simulink model "controller_hor"  (R2020b)
settings: Solver=ode45  StartTime=0.0  StopTime=2  MaxStep=0.01  RelTol=1e-3
values from neighbouring files (symbols this model uses):
  g = 9.81    [matlab.mat]
  J_xx = 400    [matlab.mat]
  J_yy = 1    [matlab.mat]
  J_zz = 400    [matlab.mat]
  k_f = 6.11e-08    [matlab.mat]
  l = 400    [matlab.mat]
  m = 1.5    [matlab.mat]
  time = 25    [matlab.mat]
  x_0 = 0    [matlab.mat]
  x_des = 6    [matlab.mat]
  y_0 = 0    [matlab.mat]
  y_des = 6    [matlab.mat]
  z_0 = 0    [matlab.mat]
  z_des = 6    [matlab.mat]
undefined symbols (not defined in the file or in its folder): k_p_fi, k_p_psi, k_p_theta, k_p_x, k_p_y, k_p_z, k_v_fi, k_v_psi, k_v_theta, k_v_x, k_v_y, k_v_z, k_X, k_Y, x_dot_min
settings Model: OrderedModelArguments=off  Creator=Danil  LastModifiedBy=Danil
settings DataIOCC: ReturnWorkspaceOutputsName=SDOSimTest_Log

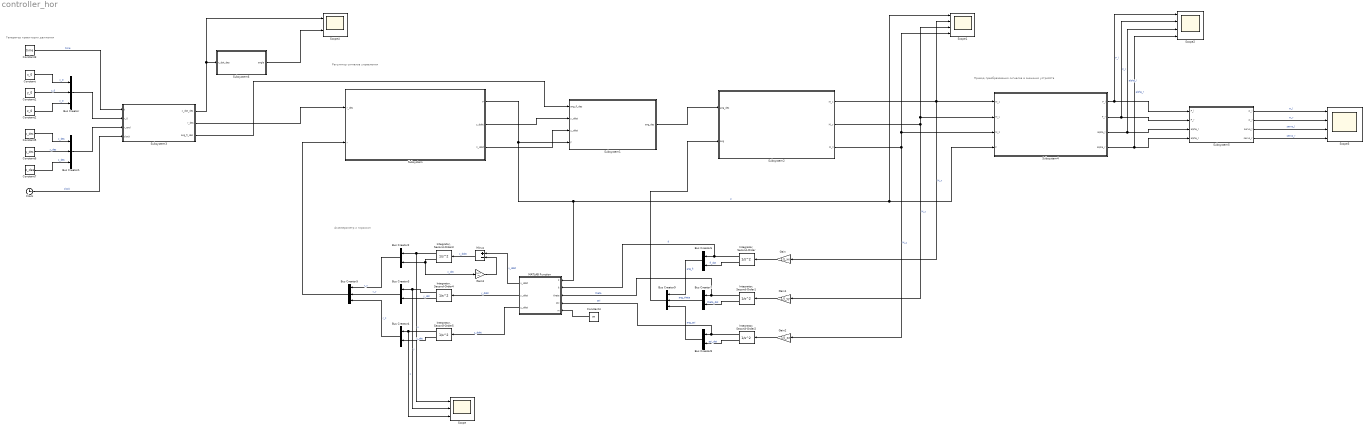
== system controller_hor ==
  note: Привод преобразования сигналов в значения устройств
  note: Регулятор сигналов управления
  note: Генератор траектории движения
  note: Акселерометр и гироскоп
  Bus Creator{,1,5,9} (4 alike) : BusCreator  Inputs=3
  Bus Creator{2..4,6..8} (6 alike) : BusCreator  Inputs=2
  Clock : Clock
  Constant : Constant  Value=x_0
  Constant1 : Constant  Value=y_0
  Constant2 : Constant  Value=z_0
  Constant3 : Constant  Value=time
  Constant4 : Constant  Value=m
  Constant5 : Constant  Value=x_des
  Constant6 : Constant  Value=y_des
  Constant7 : Constant  Value=z_des
  Gain : Gain  Gain=1/J_xx
  Gain1 : Gain  Gain=1/J_yy
  Gain2 : Gain  Gain=1/J_zz
  Gain3 : Gain  Gain=k_X / m
  Integrator, Second-Order{,1..2,4..5} (5 alike) : SecondOrderIntegrator
  "Integrator, Second-Order3" : SecondOrderIntegrator  ICDXDT=x_dot_min
  MATLAB Function : MATLAB Function  TreatAsAtomicUnit=on
  Minus : Sum  Inputs=+-
  Scope : Scope  NumInputPorts=3
  Scope1 : Scope  NumInputPorts=4
  Scope2 : Scope  NumInputPorts=4
  Scope3 : Scope  NumInputPorts=4
  Scope4 : Scope  NumInputPorts=2
  Subsystem : Subsystem
  Subsystem1 : Subsystem
  Subsystem2 : Subsystem
  Subsystem3 : Subsystem
  Subsystem4 : Subsystem
  Subsystem5 : Subsystem
  Subsystem6 : Subsystem
  wires:
  Subsystem2/2(M_y) -> Gain1/1, Subsystem4/2(M_y), Scope1/3  "M_y"
  Constant2/1 -> Bus Creator/3  "z_0"
  Subsystem5/4(servo_r) -> Scope3/4  "servo_r"
  Subsystem2/1(M_x) -> Subsystem4/1(M_x), Gain/1, Scope1/2  "M_x"
  Subsystem4/2(F_r) -> Scope2/2, Subsystem5/2(F_r)  "F_r"
  Subsystem5/3(servo_l) -> Scope3/3  "servo_l"
  Subsystem5/1(w_l) -> Scope3/1  "w_l"
  Subsystem/2(y_ddot) -> Subsystem1/2(y_ddot)
  Bus Creator6/1 -> Bus Creator9/1  "ang_fi"
  Subsystem5/2(w_r) -> Scope3/2  "w_r"
  Subsystem4/4(alpha_r) -> Scope2/4, Subsystem5/4(alpha_r)  "alpha_r"
  Constant1/1 -> Bus Creator/2  "y_0"
  Subsystem4/3(alpha_l) -> Scope2/3, Subsystem5/3(alpha_l)  "alpha_l"
  "Integrator, Second-Order2"/2 -> Bus Creator8/2  "psi_dot"
  "Integrator, Second-Order"/2 -> Bus Creator6/2  "fi_dot"
  Subsystem4/1(F_l) -> Scope2/1, Subsystem5/1(F_l)  "F_l"
  "Integrator, Second-Order3"/1 -> Scope/1, Bus Creator2/1  "x"
  "Integrator, Second-Order5"/2 -> Bus Creator4/2  "z_dot"
  Constant4/1 -> MATLAB Function/5(m)
  "Integrator, Second-Order1"/1 -> MATLAB Function/3(theta), Bus Creator7/1  "theta"
  "Integrator, Second-Order1"/2 -> Bus Creator7/2  "theta_dot"
  Subsystem/1(F) -> Subsystem1/4(F), MATLAB Function/1(F), Scope1/1, Subsystem4/4(F)  "F"
  "Integrator, Second-Order2"/1 -> MATLAB Function/4(psi), Bus Creator8/1  "psi"
  Bus Creator7/1 -> Bus Creator9/2  "ang_theta"
  Gain2/1 -> "Integrator, Second-Order2"/1
  Subsystem/3(z_ddot) -> Subsystem1/3(z_ddot)
  Constant5/1 -> Bus Creator1/1  "x_des"
  Bus Creator4/1 -> Bus Creator5/3  "r_z"
  Bus Creator3/1 -> Bus Creator5/2  "r_y"
  Subsystem2/3(M_z) -> Gain2/1, Subsystem4/3(M_z), Scope1/4  "M_z"
  "Integrator, Second-Order"/1 -> MATLAB Function/2(fi), Bus Creator6/1  "fi"
  "Integrator, Second-Order4"/1 -> Scope/2, Bus Creator3/1  "y"
  Subsystem3/2(r_des) -> Subsystem/1(r_des)
  Subsystem3/3(ang_fi_des) -> Subsystem1/1(ang_fi_des)
  Constant7/1 -> Bus Creator1/3  "z_des"
  Bus Creator/1 -> Subsystem3/2(r_0)
  Constant3/1 -> Subsystem3/1(t)  "time"
  "Integrator, Second-Order3"/2 -> Gain3/1, Bus Creator2/2  "x_dot"
  Bus Creator2/1 -> Bus Creator5/1  "r_x"
  Bus Creator5/1 -> Subsystem/2(r)
  "Integrator, Second-Order4"/2 -> Bus Creator3/2  "y_dot"
  MATLAB Function/3(z_ddot) -> "Integrator, Second-Order5"/1  "z_ddot"
  Clock/1 -> Subsystem3/4(clock)  "clock"
  Bus Creator1/1 -> Subsystem3/3(r_end)
  "Integrator, Second-Order5"/1 -> Scope/3, Bus Creator4/1  "z"
  Constant/1 -> Bus Creator/1  "x_0"
  Gain1/1 -> "Integrator, Second-Order1"/1
  MATLAB Function/2(y_ddot) -> "Integrator, Second-Order4"/1  "y_ddot"
  Bus Creator8/1 -> Bus Creator9/3  "ang_psi"
  Gain/1 -> "Integrator, Second-Order"/1
  Constant6/1 -> Bus Creator1/2  "y_des"
  Subsystem3/1(x_dot_des) -> Scope4/1, Subsystem6/1(x_dot_des)
  Subsystem1/1(ang_des) -> Subsystem2/1(ang_des)
  Bus Creator9/1 -> Subsystem2/2(ang)
  Subsystem6/1(angle) -> Scope4/2
  Minus/1 -> "Integrator, Second-Order3"/1  "x_ddot"
  MATLAB Function/1(x_ddot) -> Minus/1  "x_ddot"
  Gain3/1 -> Minus/2

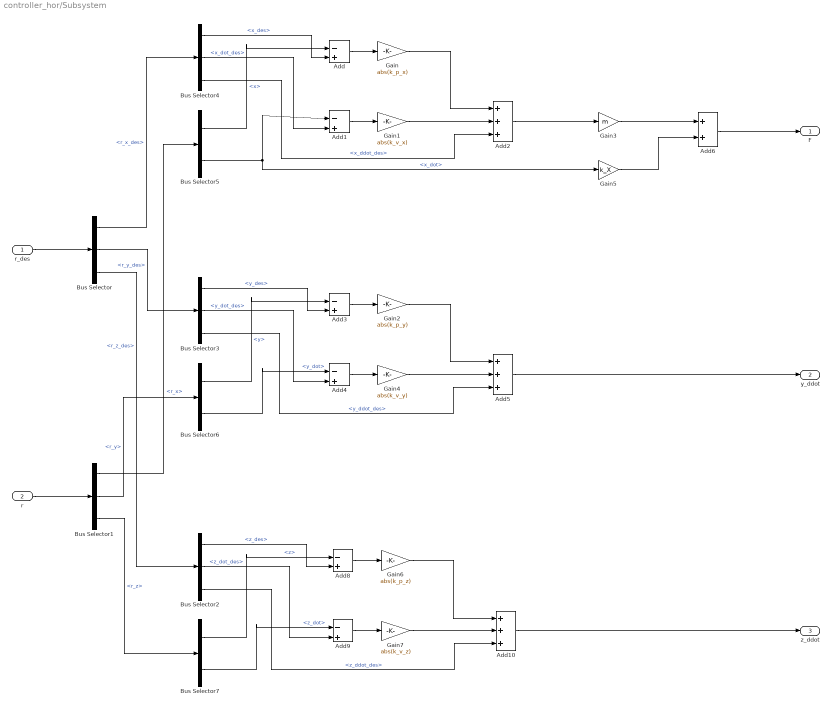
== system controller_hor/Subsystem ==
  r_des : Inport
  r : Inport  Port=2
  Add{,1,3..4,8..9} (6 alike) : Sum  Inputs=-|+
  Add10 : Sum  Inputs=+++
  Add2 : Sum  Inputs=+++
  Add5 : Sum  Inputs=+++
  Add6 : Sum
  Bus Selector : BusSelector  OutputSignals=r_x_des,r_y_des,r_z_des
  Bus Selector1 : BusSelector  OutputSignals=r_x,r_y,r_z
  Bus Selector2 : BusSelector  OutputSignals=z_des,z_dot_des,z_ddot_des
  Bus Selector3 : BusSelector  OutputSignals=y_des,y_dot_des,y_ddot_des
  Bus Selector4 : BusSelector  OutputSignals=x_des,x_dot_des,x_ddot_des
  Bus Selector5 : BusSelector  OutputSignals=x,x_dot
  Bus Selector6 : BusSelector  OutputSignals=y,y_dot
  Bus Selector7 : BusSelector  OutputSignals=z,z_dot
  Gain : Gain  Gain=abs(k_p_x)
  Gain1 : Gain  Gain=abs(k_v_x)
  Gain2 : Gain  Gain=abs(k_p_y)
  Gain3 : Gain  Gain=m
  Gain4 : Gain  Gain=abs(k_v_y)
  Gain5 : Gain  Gain=k_X
  Gain6 : Gain  Gain=abs(k_p_z)
  Gain7 : Gain  Gain=abs(k_v_z)
  F : Outport
  y_ddot : Outport  Port=2
  z_ddot : Outport  Port=3
  wires:
  Gain/1 -> Add2/1
  Add/1 -> Gain/1
  Add1/1 -> Gain1/1
  Gain1/1 -> Add2/2
  Add4/1 -> Gain4/1
  Add5/1 -> y_ddot/1
  Gain4/1 -> Add5/2
  Gain2/1 -> Add5/1
  Add3/1 -> Gain2/1
  Add9/1 -> Gain7/1
  Gain7/1 -> Add10/2
  Gain6/1 -> Add10/1
  Add8/1 -> Gain6/1
  Add10/1 -> z_ddot/1
  r_des/1 -> Bus Selector/1
  r/1 -> Bus Selector1/1
  Bus Selector4/1 -> Add/2  "<x_des>"
  Bus Selector4/2 -> Add1/2  "<x_dot_des>"
  Bus Selector4/3 -> Add2/3  "<x_ddot_des>"
  Bus Selector5/1 -> Add/1  "<x>"
  Bus Selector5/2 -> Gain5/1, Add1/1  "<x_dot>"
  Bus Selector3/1 -> Add3/2  "<y_des>"
  Bus Selector3/2 -> Add4/2  "<y_dot_des>"
  Bus Selector3/3 -> Add5/3  "<y_ddot_des>"
  Bus Selector6/1 -> Add3/1  "<y>"
  Bus Selector6/2 -> Add4/1  "<y_dot>"
  Bus Selector2/1 -> Add8/2  "<z_des>"
  Bus Selector2/2 -> Add9/2  "<z_dot_des>"
  Bus Selector2/3 -> Add10/3  "<z_ddot_des>"
  Bus Selector7/1 -> Add8/1  "<z>"
  Bus Selector7/2 -> Add9/1  "<z_dot>"
  Bus Selector/1 -> Bus Selector4/1  "<r_x_des>"
  Bus Selector/2 -> Bus Selector3/1  "<r_y_des>"
  Bus Selector/3 -> Bus Selector2/1  "<r_z_des>"
  Bus Selector1/1 -> Bus Selector5/1  "<r_x>"
  Bus Selector1/2 -> Bus Selector6/1  "<r_y>"
  Bus Selector1/3 -> Bus Selector7/1  "<r_z>"
  Add2/1 -> Gain3/1
  Gain3/1 -> Add6/1
  Add6/1 -> F/1
  Gain5/1 -> Add6/2

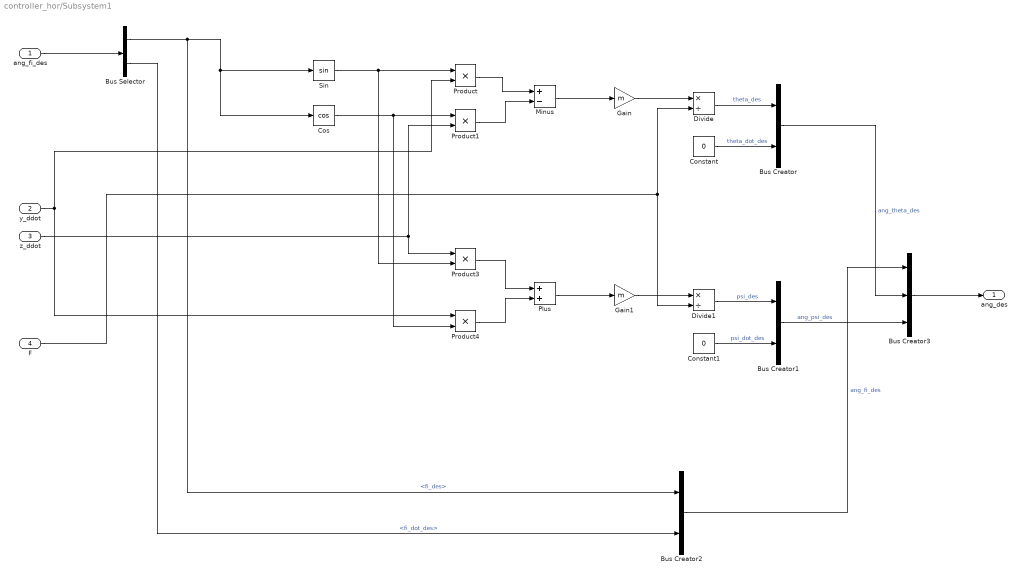
== system controller_hor/Subsystem1 ==
  ang_fi_des : Inport
  y_ddot : Inport  Port=2
  z_ddot : Inport  Port=3
  F : Inport  Port=4
  Bus Creator : BusCreator  Inputs=2
  Bus Creator1 : BusCreator  Inputs=2
  Bus Creator2 : BusCreator  Inputs=2
  Bus Creator3 : BusCreator  Inputs=3
  Bus Selector : BusSelector  OutputSignals=fi_des,fi_dot_des
  Constant : Constant  Value=0
  Constant1 : Constant  Value=0
  Cos : Trigonometry  Operator=cos
  Divide : Product  Inputs=*/
  Divide1 : Product  Inputs=*/
  Gain : Gain  Gain=m
  Gain1 : Gain  Gain=m
  Minus : Sum  Inputs=+-
  Plus : Sum
  Product{,1,3..4} (4 alike) : Product
  Sin : Trigonometry
  ang_des : Outport
  wires:
  Sin/1 -> Product3/2, Product/1
  Product1/1 -> Minus/2
  Product/1 -> Minus/1
  z_ddot/1 -> Product1/2, Product3/1
  Cos/1 -> Product4/2, Product1/1
  y_ddot/1 -> Product/2, Product4/1
  Product4/1 -> Plus/2
  Product3/1 -> Plus/1
  ang_fi_des/1 -> Bus Selector/1
  Bus Selector/1 -> Bus Creator2/1, Sin/1, Cos/1  "<fi_des>"
  Bus Selector/2 -> Bus Creator2/2  "<fi_dot_des>"
  Constant/1 -> Bus Creator/2  "theta_dot_des"
  Constant1/1 -> Bus Creator1/2  "psi_dot_des"
  Bus Creator3/1 -> ang_des/1
  Bus Creator2/1 -> Bus Creator3/1  "ang_fi_des"
  Minus/1 -> Gain/1
  Gain/1 -> Divide/1
  F/1 -> Divide/2, Divide1/2
  Divide/1 -> Bus Creator/1  "theta_des"
  Plus/1 -> Gain1/1
  Gain1/1 -> Divide1/1
  Divide1/1 -> Bus Creator1/1  "psi_des"
  Bus Creator/1 -> Bus Creator3/2  "ang_theta_des"
  Bus Creator1/1 -> Bus Creator3/3  "ang_psi_des"

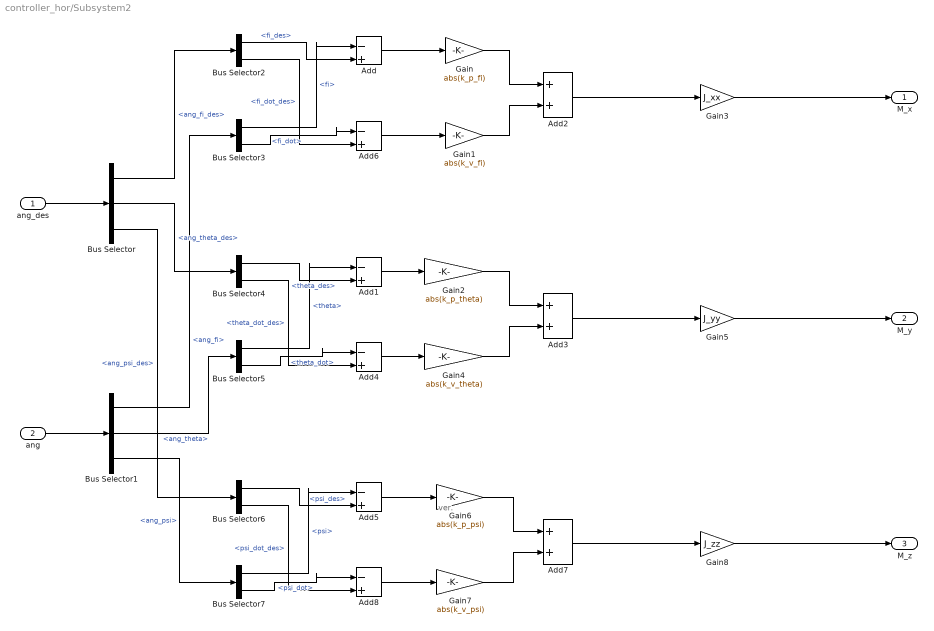
== system controller_hor/Subsystem2 ==
  note: ver.
  ang_des : Inport
  ang : Inport  Port=2
  Add{,1,4..6,8} (6 alike) : Sum  Inputs=-|+
  Add2 : Sum
  Add3 : Sum
  Add7 : Sum
  Bus Selector : BusSelector  OutputSignals=ang_fi_des,ang_theta_des,ang_psi_des
  Bus Selector1 : BusSelector  OutputSignals=ang_fi,ang_theta,ang_psi
  Bus Selector2 : BusSelector  OutputSignals=fi_des,fi_dot_des
  Bus Selector3 : BusSelector  OutputSignals=fi,fi_dot
  Bus Selector4 : BusSelector  OutputSignals=theta_des,theta_dot_des
  Bus Selector5 : BusSelector  OutputSignals=theta,theta_dot
  Bus Selector6 : BusSelector  OutputSignals=psi_des,psi_dot_des
  Bus Selector7 : BusSelector  OutputSignals=psi,psi_dot
  Gain : Gain  Gain=abs(k_p_fi)
  Gain1 : Gain  Gain=abs(k_v_fi)
  Gain2 : Gain  Gain=abs(k_p_theta)
  Gain3 : Gain  Gain=J_xx
  Gain4 : Gain  Gain=abs(k_v_theta)
  Gain5 : Gain  Gain=J_yy
  Gain6 : Gain  Gain=abs(k_p_psi)
  Gain7 : Gain  Gain=abs(k_v_psi)
  Gain8 : Gain  Gain=J_zz
  M_x : Outport
  M_y : Outport  Port=2
  M_z : Outport  Port=3
  wires:
  Gain/1 -> Add2/1
  Gain1/1 -> Add2/2
  Add/1 -> Gain/1
  Add2/1 -> Gain3/1
  Gain3/1 -> M_x/1
  Add6/1 -> Gain1/1
  Add1/1 -> Gain2/1
  Gain5/1 -> M_y/1
  Add3/1 -> Gain5/1
  Gain2/1 -> Add3/1
  Gain4/1 -> Add3/2
  Add4/1 -> Gain4/1
  Add5/1 -> Gain6/1
  Gain8/1 -> M_z/1
  Add7/1 -> Gain8/1
  Gain6/1 -> Add7/1
  Gain7/1 -> Add7/2
  Add8/1 -> Gain7/1
  ang_des/1 -> Bus Selector/1
  ang/1 -> Bus Selector1/1
  Bus Selector2/1 -> Add/2  "<fi_des>"
  Bus Selector3/1 -> Add/1  "<fi>"
  Bus Selector2/2 -> Add6/2  "<fi_dot_des>"
  Bus Selector3/2 -> Add6/1  "<fi_dot>"
  Bus Selector4/1 -> Add1/2  "<theta_des>"
  Bus Selector5/1 -> Add1/1  "<theta>"
  Bus Selector4/2 -> Add4/2  "<theta_dot_des>"
  Bus Selector5/2 -> Add4/1  "<theta_dot>"
  Bus Selector6/1 -> Add5/2  "<psi_des>"
  Bus Selector7/1 -> Add5/1  "<psi>"
  Bus Selector6/2 -> Add8/2  "<psi_dot_des>"
  Bus Selector7/2 -> Add8/1  "<psi_dot>"
  Bus Selector/1 -> Bus Selector2/1  "<ang_fi_des>"
  Bus Selector/2 -> Bus Selector4/1  "<ang_theta_des>"
  Bus Selector/3 -> Bus Selector6/1  "<ang_psi_des>"
  Bus Selector1/1 -> Bus Selector3/1  "<ang_fi>"
  Bus Selector1/2 -> Bus Selector5/1  "<ang_theta>"
  Bus Selector1/3 -> Bus Selector7/1  "<ang_psi>"

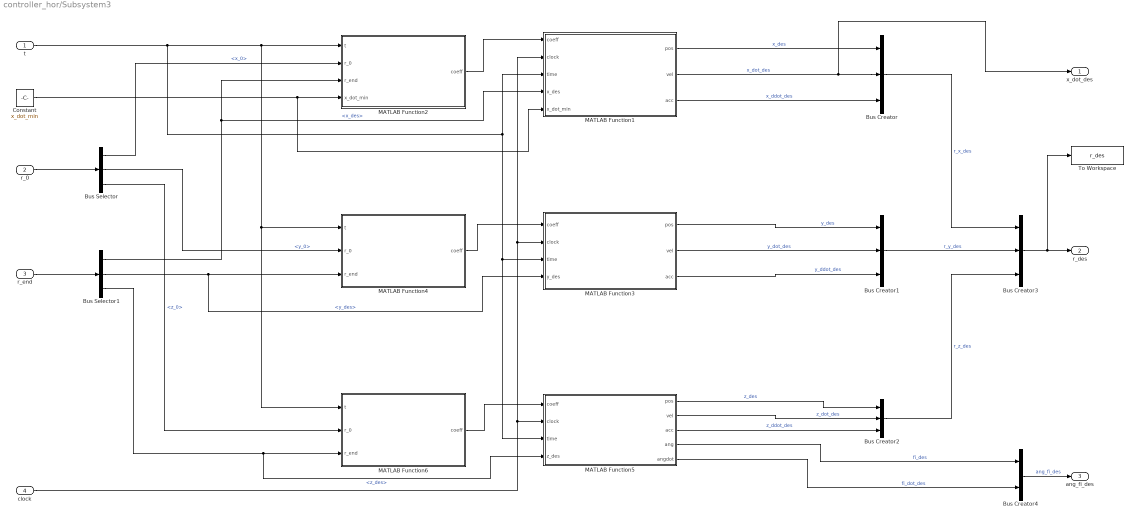
== system controller_hor/Subsystem3 ==
  t : Inport
  r_0 : Inport  Port=2
  r_end : Inport  Port=3
  clock : Inport  Port=4
  Bus Creator{,1..3} (4 alike) : BusCreator  Inputs=3
  Bus Creator4 : BusCreator  Inputs=2
  Bus Selector : BusSelector  OutputSignals=x_0,y_0,z_0
  Bus Selector1 : BusSelector  OutputSignals=x_des,y_des,z_des
  Constant : Constant  Value=x_dot_min
  MATLAB Function1 : MATLAB Function  TreatAsAtomicUnit=on
  MATLAB Function2 : MATLAB Function  TreatAsAtomicUnit=on
  MATLAB Function3 : MATLAB Function  TreatAsAtomicUnit=on
  MATLAB Function4 : MATLAB Function  TreatAsAtomicUnit=on
  MATLAB Function5 : MATLAB Function  TreatAsAtomicUnit=on
  MATLAB Function6 : MATLAB Function  TreatAsAtomicUnit=on
  To Workspace : ToWorkspace  VariableName=r_des  SaveFormat=Timeseries  SampleTime=-1
  x_dot_des : Outport
  r_des : Outport  Port=2
  ang_fi_des : Outport  Port=3
  wires:
  MATLAB Function2/1(coeff) -> MATLAB Function1/1(coeff)
  MATLAB Function4/1(coeff) -> MATLAB Function3/1(coeff)
  MATLAB Function6/1(coeff) -> MATLAB Function5/1(coeff)
  t/1 -> MATLAB Function5/3(time), MATLAB Function3/3(time), MATLAB Function1/3(time), MATLAB Function6/1(t), MATLAB Function4/1(t), MATLAB Function2/1(t)
  clock/1 -> MATLAB Function1/2(clock), MATLAB Function3/2(clock), MATLAB Function5/2(clock)
  r_0/1 -> Bus Selector/1
  r_end/1 -> Bus Selector1/1
  Bus Selector/1 -> MATLAB Function2/2(r_0)  "<x_0>"
  Bus Selector/2 -> MATLAB Function4/2(r_0)  "<y_0>"
  Bus Selector/3 -> MATLAB Function6/2(r_0)  "<z_0>"
  Bus Selector1/1 -> MATLAB Function1/4(x_des), MATLAB Function2/3(r_end)  "<x_des>"
  Bus Selector1/2 -> MATLAB Function3/4(y_des), MATLAB Function4/3(r_end)  "<y_des>"
  Bus Selector1/3 -> MATLAB Function5/4(z_des), MATLAB Function6/3(r_end)  "<z_des>"
  MATLAB Function1/1(pos) -> Bus Creator/1  "x_des"
  MATLAB Function1/2(vel) -> x_dot_des/1, Bus Creator/2  "x_dot_des"
  MATLAB Function1/3(acc) -> Bus Creator/3  "x_ddot_des"
  MATLAB Function3/1(pos) -> Bus Creator1/1  "y_des"
  MATLAB Function3/2(vel) -> Bus Creator1/2  "y_dot_des"
  MATLAB Function3/3(acc) -> Bus Creator1/3  "y_ddot_des"
  MATLAB Function5/1(pos) -> Bus Creator2/1  "z_des"
  MATLAB Function5/2(vel) -> Bus Creator2/2  "z_dot_des"
  MATLAB Function5/3(acc) -> Bus Creator2/3  "z_ddot_des"
  MATLAB Function5/4(ang) -> Bus Creator4/1  "fi_des"
  MATLAB Function5/5(angdot) -> Bus Creator4/2  "fi_dot_des"
  Bus Creator/1 -> Bus Creator3/1  "r_x_des"
  Bus Creator1/1 -> Bus Creator3/2  "r_y_des"
  Bus Creator2/1 -> Bus Creator3/3  "r_z_des"
  Bus Creator3/1 -> To Workspace/1, r_des/1
  Bus Creator4/1 -> ang_fi_des/1  "ang_fi_des"
  Constant/1 -> MATLAB Function1/5(x_dot_min), MATLAB Function2/4(x_dot_min)

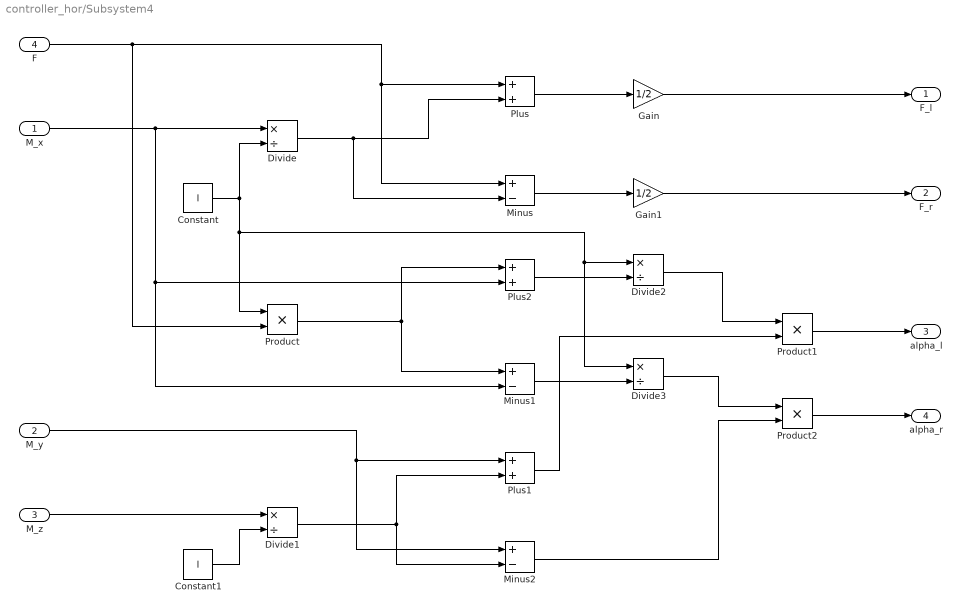
== system controller_hor/Subsystem4 ==
  M_x : Inport
  M_y : Inport  Port=2
  M_z : Inport  Port=3
  F : Inport  Port=4
  Constant : Constant  Value=l
  Constant1 : Constant  Value=l
  Divide{,1..3} (4 alike) : Product  Inputs=*/
  Gain : Gain  Gain=1/2
  Gain1 : Gain  Gain=1/2
  Minus : Sum  Inputs=+-
  Minus1 : Sum  Inputs=+-
  Minus2 : Sum  Inputs=+-
  Plus : Sum
  Plus1 : Sum
  Plus2 : Sum
  Product : Product
  Product1 : Product
  Product2 : Product
  F_l : Outport
  F_r : Outport  Port=2
  alpha_l : Outport  Port=3
  alpha_r : Outport  Port=4
  wires:
  M_x/1 -> Minus1/2, Plus2/2, Divide/1
  Constant/1 -> Divide3/1, Divide2/1, Product/1, Divide/2
  F/1 -> Product/2, Minus/1, Plus/1
  Divide/1 -> Minus/2, Plus/2
  Plus/1 -> Gain/1
  Gain/1 -> F_l/1
  Minus/1 -> Gain1/1
  Gain1/1 -> F_r/1
  M_z/1 -> Divide1/1
  Constant1/1 -> Divide1/2
  M_y/1 -> Minus2/1, Plus1/1
  Divide1/1 -> Minus2/2, Plus1/2
  Product/1 -> Minus1/1, Plus2/1
  Plus2/1 -> Divide2/2
  Minus1/1 -> Divide3/2
  Divide2/1 -> Product1/1
  Plus1/1 -> Product1/2
  Product1/1 -> alpha_l/1
  Product2/1 -> alpha_r/1
  Divide3/1 -> Product2/1
  Minus2/1 -> Product2/2

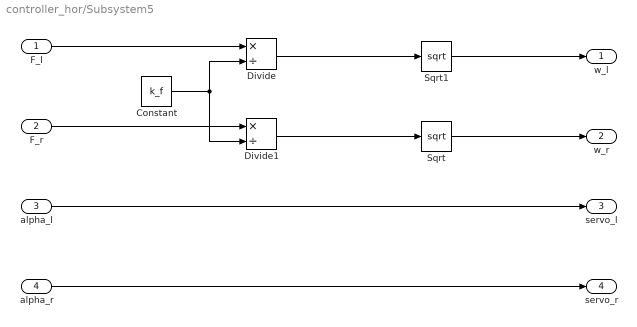
== system controller_hor/Subsystem5 ==
  F_l : Inport
  F_r : Inport  Port=2
  alpha_l : Inport  Port=3
  alpha_r : Inport  Port=4
  Constant : Constant  Value=k_f
  Divide : Product  Inputs=*/
  Divide1 : Product  Inputs=*/
  Sqrt : Sqrt  SaturateOnIntegerOverflow=on
  Sqrt1 : Sqrt  SaturateOnIntegerOverflow=on
  w_l : Outport
  w_r : Outport  Port=2
  servo_l : Outport  Port=3
  servo_r : Outport  Port=4
  wires:
  alpha_l/1 -> servo_l/1
  alpha_r/1 -> servo_r/1
  Sqrt/1 -> w_r/1
  Sqrt1/1 -> w_l/1
  F_l/1 -> Divide/1
  F_r/1 -> Divide1/1
  Constant/1 -> Divide1/2, Divide/2
  Divide/1 -> Sqrt1/1
  Divide1/1 -> Sqrt/1

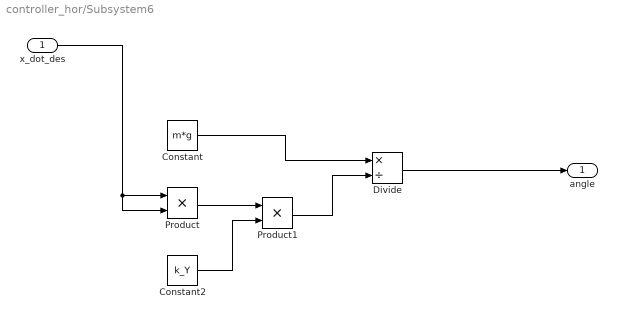
== system controller_hor/Subsystem6 ==
  x_dot_des : Inport
  Constant : Constant  Value=m*g
  Constant2 : Constant  Value=k_Y
  Divide : Product  Inputs=*/
  Product : Product
  Product1 : Product
  angle : Outport
  wires:
  x_dot_des/1 -> Product/2, Product/1
  Constant/1 -> Divide/1
  Constant2/1 -> Product1/2
  Divide/1 -> angle/1
  Product/1 -> Product1/1
  Product1/1 -> Divide/2

== matlab function controller_hor/Subsystem3/MATLAB Function1 ==
  data: coeff input; pos output; clock input; vel output; acc output; time input; x_des input; x_dot_min input
function [pos, vel, acc] = trajectories_calculation(coeff, clock, time, x_des, x_dot_min)

T_p = [clock^5      clock^4     clock^3     clock^2     clock   1]';
T_v = [5*clock^4    4*clock^3   3*clock^2   2*clock     1       0]';
T_a = [20*clock^3   12*clock^2  6*clock     2           0       0]';

pos = sum(coeff.*T_p);
vel = sum(coeff.*T_v);
acc = sum(coeff.*T_a);

if clock >= time
    pos = x_des + x_dot_min * (clock - time);
    vel = x_dot_min;
    acc = 0;
end

== matlab function controller_hor/MATLAB Function ==
  data: x_ddot output; y_ddot output; F input; fi input; theta input; psi input; z_ddot output; m input
function [x_ddot, y_ddot, z_ddot] = sensors(F, fi, theta, psi, m)

a = F / m;

R_x_fi = [1 0 0; 0 cos(fi) -sin(fi); 0 sin(fi) cos(fi)];
R_y_theta = [cos(theta) 0 sin(theta); 0 1 0; -sin(theta) 0 cos(theta)];
R_z_psi = [cos(psi) -sin(psi) 0; sin(psi) cos(psi) 0; 0 0 1];

R_xyz = R_x_fi * R_y_theta * R_z_psi;

x_ddot = R_xyz(1, 1) * a;
y_ddot = R_xyz(2, 1) * a;
z_ddot = R_xyz(3, 1) * a;

== matlab function controller_hor/Subsystem3/MATLAB Function2 ==
  data: t input; coeff output; r_0 input; r_end input; x_dot_min input
function coeff  = calculation_coefficients(t, r_0, r_end, x_dot_min)

x_0 = r_0;
x_dot_0 = x_dot_min;
x_ddot_0 = 0;

x_des = r_end;
x_dot_des = x_dot_min;
x_ddot_des = 0;

waypoints = [x_0    x_dot_0     x_ddot_0;
             x_des  x_dot_des   x_ddot_des]';
t = [0 t];

time_size = size(t);
n = 0;
%T = linspace(0, time_size(2) - 1, point(2));


border_conditions_sigm = reshape(waypoints(:, n + 1 : n + 2),1,[]);
%disp(border_conditions_sigm)

coeff = zeros(6, 1);

parameters = [1 * (t(n + 1) ^ 5), 1 * (t(n + 1) ^ 4), 1 * (t(n + 1) ^ 3), 1 * (t(n + 1) ^ 2), 1 * (t(n + 1) ^ 1), 1 * (t(n + 1) ^ 0);
              5 * (t(n + 1) ^ 4), 4 * (t(n + 1) ^ 3), 3 * (t(n + 1) ^ 2), 2 * (t(n + 1) ^ 1), 1 * (t(n + 1) ^ 0), 0 * (t(n + 1) ^ 0);
              20 * (t(n + 1) ^ 3), 12 * (t(n + 1) ^ 2), 6 * (t(n + 1) ^ 1), 2 * (t(n + 1) ^ 0), 0 * (t(n + 1) ^ 0), 0 * (t(n + 1) ^ 0);
              1 * (t(n + 2) ^ 5), 1 * (t(n + 2) ^ 4), 1 * (t(n + 2) ^ 3), 1 * (t(n + 2) ^ 2), 1 * (t(n + 2) ^ 1), 1 * (t(n + 2) ^ 0);
              5 * (t(n + 2) ^ 4), 4 * (t(n + 2) ^ 3), 3 * (t(n + 2) ^ 2), 2 * (t(n + 2) ^ 1), 1 * (t(n + 2) ^ 0), 0 * (t(n + 2) ^ 0);
              20 * (t(n + 2) ^ 3), 12 * (t(n + 2) ^ 2), 6 * (t(n + 2) ^ 1), 2 * (t(n + 2) ^ 0), 0 * (t(n + 2) ^ 0), 0 * (t(n + 2) ^ 0)];

coeff = inv(parameters) * border_conditions_sigm';

== matlab function controller_hor/Subsystem3/MATLAB Function3 ==
  data: coeff input; pos output; clock input; vel output; acc output; time input; y_des input
function [pos, vel, acc] = trajectories_calculation(coeff, clock, time, y_des)

T_p = [clock^5      clock^4     clock^3     clock^2     clock   1]';
T_v = [5*clock^4    4*clock^3   3*clock^2   2*clock     1       0]';
T_a = [20*clock^3   12*clock^2  6*clock     2           0       0]';

pos = sum(coeff.*T_p);
vel = sum(coeff.*T_v);
acc = sum(coeff.*T_a);

if clock >= time
    pos = y_des;
    vel = 0;
    acc = 0;
end

== matlab function controller_hor/Subsystem3/MATLAB Function4 ==
  data: t input; coeff output; r_0 input; r_end input
function coeff  = calculation_coefficients(t, r_0, r_end)

x_0 = r_0;
x_dot_0 = 0;
x_ddot_0 = 0;

x_des = r_end;
x_dot_des = 0;
x_ddot_des = 0;

waypoints = [x_0    x_dot_0     x_ddot_0;
             x_des  x_dot_des   x_ddot_des]';
t = [0 t];

time_size = size(t);
n = 0;
%T = linspace(0, time_size(2) - 1, point(2));


border_conditions_sigm = reshape(waypoints(:, n + 1 : n + 2),1,[]);
%disp(border_conditions_sigm)

coeff = zeros(6, 1);

parameters = [1 * (t(n + 1) ^ 5), 1 * (t(n + 1) ^ 4), 1 * (t(n + 1) ^ 3), 1 * (t(n + 1) ^ 2), 1 * (t(n + 1) ^ 1), 1 * (t(n + 1) ^ 0);
              5 * (t(n + 1) ^ 4), 4 * (t(n + 1) ^ 3), 3 * (t(n + 1) ^ 2), 2 * (t(n + 1) ^ 1), 1 * (t(n + 1) ^ 0), 0 * (t(n + 1) ^ 0);
              20 * (t(n + 1) ^ 3), 12 * (t(n + 1) ^ 2), 6 * (t(n + 1) ^ 1), 2 * (t(n + 1) ^ 0), 0 * (t(n + 1) ^ 0), 0 * (t(n + 1) ^ 0);
              1 * (t(n + 2) ^ 5), 1 * (t(n + 2) ^ 4), 1 * (t(n + 2) ^ 3), 1 * (t(n + 2) ^ 2), 1 * (t(n + 2) ^ 1), 1 * (t(n + 2) ^ 0);
              5 * (t(n + 2) ^ 4), 4 * (t(n + 2) ^ 3), 3 * (t(n + 2) ^ 2), 2 * (t(n + 2) ^ 1), 1 * (t(n + 2) ^ 0), 0 * (t(n + 2) ^ 0);
              20 * (t(n + 2) ^ 3), 12 * (t(n + 2) ^ 2), 6 * (t(n + 2) ^ 1), 2 * (t(n + 2) ^ 0), 0 * (t(n + 2) ^ 0), 0 * (t(n + 2) ^ 0)];

coeff = inv(parameters) * border_conditions_sigm';

== matlab function controller_hor/Subsystem3/MATLAB Function5 ==
  data: coeff input; pos output; clock input; vel output; acc output; ang output; angdot output; time input; z_des input
function [pos, vel, acc, ang, angdot] = trajectories_calculation(coeff, clock, time, z_des)

T_p = [clock^5      clock^4     clock^3     clock^2     clock   1]';
T_v = [5*clock^4    4*clock^3   3*clock^2   2*clock     1       0]';
T_a = [20*clock^3   12*clock^2  6*clock     2           0       0]';

pos = sum(coeff.*T_p);
vel = sum(coeff.*T_v);
acc = sum(coeff.*T_a);
ang = 0;
angdot = 0;

if clock >= time
    pos = z_des;
    vel = 0;
    acc = 0;
end

== matlab function controller_hor/Subsystem3/MATLAB Function6 ==
  data: t input; coeff output; r_0 input; r_end input
function coeff  = calculation_coefficients(t, r_0, r_end)

x_0 = r_0;
x_dot_0 = 0;
x_ddot_0 = 0;

x_des = r_end;
x_dot_des = 0;
x_ddot_des = 0;

waypoints = [x_0    x_dot_0     x_ddot_0;
             x_des  x_dot_des   x_ddot_des]';
t = [0 t];

time_size = size(t);
n = 0;
%T = linspace(0, time_size(2) - 1, point(2));


border_conditions_sigm = reshape(waypoints(:, n + 1 : n + 2),1,[]);
%disp(border_conditions_sigm)

coeff = zeros(6, 1);

parameters = [1 * (t(n + 1) ^ 5), 1 * (t(n + 1) ^ 4), 1 * (t(n + 1) ^ 3), 1 * (t(n + 1) ^ 2), 1 * (t(n + 1) ^ 1), 1 * (t(n + 1) ^ 0);
              5 * (t(n + 1) ^ 4), 4 * (t(n + 1) ^ 3), 3 * (t(n + 1) ^ 2), 2 * (t(n + 1) ^ 1), 1 * (t(n + 1) ^ 0), 0 * (t(n + 1) ^ 0);
              20 * (t(n + 1) ^ 3), 12 * (t(n + 1) ^ 2), 6 * (t(n + 1) ^ 1), 2 * (t(n + 1) ^ 0), 0 * (t(n + 1) ^ 0), 0 * (t(n + 1) ^ 0);
              1 * (t(n + 2) ^ 5), 1 * (t(n + 2) ^ 4), 1 * (t(n + 2) ^ 3), 1 * (t(n + 2) ^ 2), 1 * (t(n + 2) ^ 1), 1 * (t(n + 2) ^ 0);
              5 * (t(n + 2) ^ 4), 4 * (t(n + 2) ^ 3), 3 * (t(n + 2) ^ 2), 2 * (t(n + 2) ^ 1), 1 * (t(n + 2) ^ 0), 0 * (t(n + 2) ^ 0);
              20 * (t(n + 2) ^ 3), 12 * (t(n + 2) ^ 2), 6 * (t(n + 2) ^ 1), 2 * (t(n + 2) ^ 0), 0 * (t(n + 2) ^ 0), 0 * (t(n + 2) ^ 0)];

coeff = inv(parameters) * border_conditions_sigm';
